simulink model "IP_TEST_MIO16E4_2015a"  (R2015a)
settings: Solver=ode3  StartTime=0.0  StopTime=200  RelTol=1e-3
undefined symbols (not defined in the file or in its folder): MIO, National_Instruments, PCI
libraries: sldrtlib x3
settings Model: SimulationMode=external  ExtModeTrigDuration=100000  Creator=Alunos  LastModifiedBy=Alunos
settings HardwareCC: ProdIntDivRoundTo=Zero  ProdEndianess=LittleEndian  ProdHWDeviceType=Intel->x86/Pentium  TargetIntDivRoundTo=Zero  TargetEndianess=LittleEndian  TargetHWDeviceType=Intel->x86/Pentium
settings RTWCC: SystemTargetFile=rtwin.tlc  TemplateMakefile=rtwin.tmf  Description=Simulink Desktop Real-Time  RTWCompilerOptimization=on
settings CodeAppCC: MaxIdLength=95
settings RTWinTargetCC: TargetPreCompLibLocation=C:\Program Files\MATLAB\R2015a\toolbox\sldrt\lib\win32

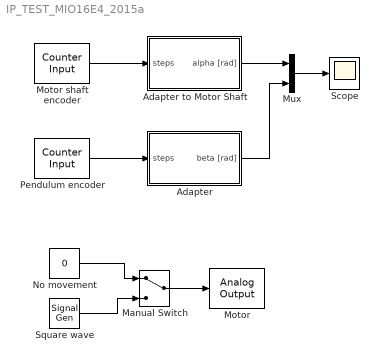
== system IP_TEST_MIO16E4_2015a ==
  Adapter : Subsystem
  Adapter to Motor Shaft : Subsystem
  Manual Switch : ManualSwitch
  Motor : sldrtlib/Analog Output  SampleTime=0.01  MaxMissedTicks=10  ShowMissedTicks=off  YieldWhenWaiting=off  DrvName=National_Instruments/PCI-MIO-16E-4  DrvAddress=4294967295  DrvOptions=[0 0 0 0 1 0]  Channels=1  RangeMode=1  VoltRange=1  InitialValue=0  FinalValue=0
      settings: AttributesFormatString=National Instruments\nPCI-MIO-16E-4 [auto]
  Motor shaft encoder : sldrtlib/Counter Input  SampleTime=0.01  MaxMissedTicks=10  ShowMissedTicks=off  YieldWhenWaiting=off  DrvName=National_Instruments/PCI-MIO-16E-4  DrvAddress=4294967295  DrvOptions=[0 0 0 0 1 0]  Channels=1  ResetMode=1  CounterEdge=1  CounterGate=1  DataType=1
      settings: AttributesFormatString=National Instruments\nPCI-MIO-16E-4 [auto]
  Mux : Mux  Inputs=2
  No movement : Constant  Value=0
  Pendulum encoder : sldrtlib/Counter Input  SampleTime=0.01  MaxMissedTicks=10  ShowMissedTicks=off  YieldWhenWaiting=off  DrvName=National_Instruments/PCI-MIO-16E-4  DrvAddress=4294967295  DrvOptions=[0 0 0 0 1 0]  Channels=2  ResetMode=1  CounterEdge=1  CounterGate=1  DataType=1
      settings: AttributesFormatString=National Instruments\nPCI-MIO-16E-4 [auto]
  Scope : Scope
      settings: YMin=-5.5  YMax=5.5
  Square wave : SignalGenerator  WaveForm=square  Frequency=.25
  wires:
  Mux/1 -> Scope/1
  Manual Switch/1 -> Motor/1
  No movement/1 -> Manual Switch/1
  Square wave/1 -> Manual Switch/2
  Pendulum encoder/1 -> Adapter/1(steps)
  Adapter/1(beta [rad]) -> Mux/2
  Motor shaft encoder/1 -> Adapter to Motor Shaft/1(steps)
  Adapter to Motor Shaft/1(alpha [rad]) -> Mux/1

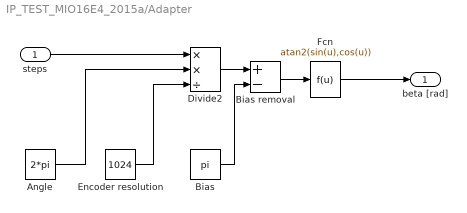
== system IP_TEST_MIO16E4_2015a/Adapter ==
  steps : Inport
  Angle : Constant  Value=2*pi
  Bias : Constant  Value=pi
  Bias removal : Sum  Inputs=+-
  Divide2 : Product  Inputs=**/
  Encoder resolution : Constant  Value=1024
  Fcn : Fcn  Expr=atan2(sin(u),cos(u))
  beta [rad] : Outport
  wires:
  Angle/1 -> Divide2/2
  Encoder resolution/1 -> Divide2/3
  steps/1 -> Divide2/1
  Bias removal/1 -> Fcn/1
  Bias/1 -> Bias removal/2
  Divide2/1 -> Bias removal/1
  Fcn/1 -> beta [rad]/1

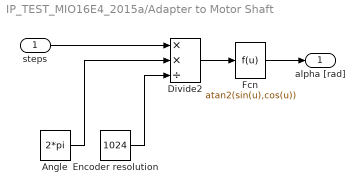
== system IP_TEST_MIO16E4_2015a/Adapter to Motor Shaft ==
  steps : Inport
  Angle : Constant  Value=2*pi
  Divide2 : Product  Inputs=**/
  Encoder resolution : Constant  Value=1024
  Fcn : Fcn  Expr=atan2(sin(u),cos(u))
  alpha [rad] : Outport
  wires:
  Angle/1 -> Divide2/2
  Encoder resolution/1 -> Divide2/3
  steps/1 -> Divide2/1
  Divide2/1 -> Fcn/1
  Fcn/1 -> alpha [rad]/1
